simulink model "IOControls"  (R2019b)
settings: configuration reference "ConfigSet_IOControls_Reference" (kept outside this file)
model workspace (MAT data in the model file):
  SampleTime = 0.05
libraries: IOStateMachinesLib x274, SignalGeneratorsLib x1, simulink x1
(part 4 of 10)

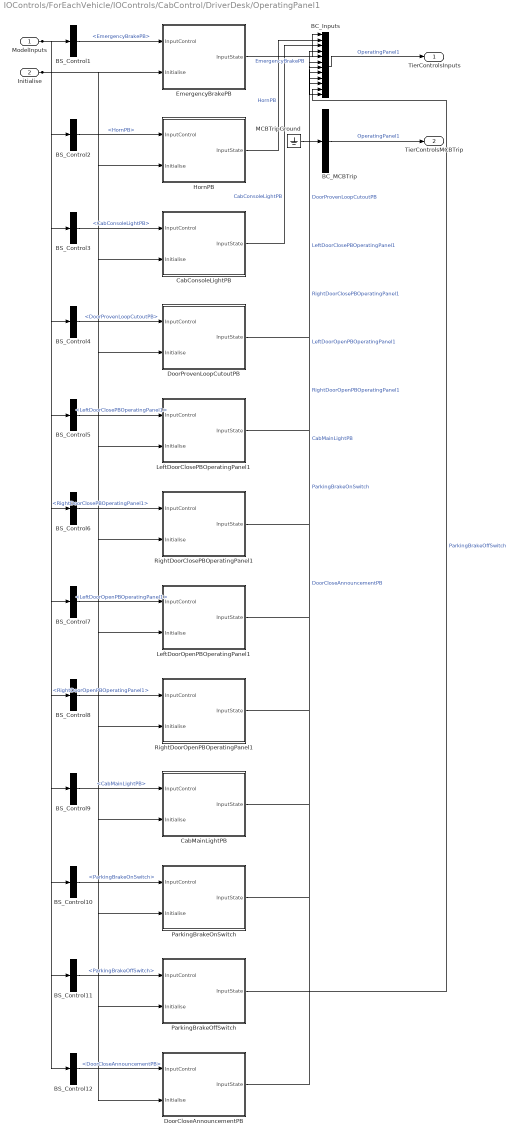
== system IOControls/ForEachVehicle/IOControls/CabControl/DriverDesk/OperatingPanel1 ==
  ModelInputs : Inport
  Initialise : Inport  Port=2
  BC_Inputs : BusCreator  Inputs=12
  BC_MCBTrip : BusCreator  Inputs=1
  BS_Control1 : BusSelector  OutputSignals=EmergencyBrakePB
  BS_Control10 : BusSelector  OutputSignals=ParkingBrakeOnSwitch
  BS_Control11 : BusSelector  OutputSignals=ParkingBrakeOffSwitch
  BS_Control12 : BusSelector  OutputSignals=DoorCloseAnnouncementPB
  BS_Control2 : BusSelector  OutputSignals=HornPB
  BS_Control3 : BusSelector  OutputSignals=CabConsoleLightPB
  BS_Control4 : BusSelector  OutputSignals=DoorProvenLoopCutoutPB
  BS_Control5 : BusSelector  OutputSignals=LeftDoorClosePBOperatingPanel1
  BS_Control6 : BusSelector  OutputSignals=RightDoorClosePBOperatingPanel1
  BS_Control7 : BusSelector  OutputSignals=LeftDoorOpenPBOperatingPanel1
  BS_Control8 : BusSelector  OutputSignals=RightDoorOpenPBOperatingPanel1
  BS_Control9 : BusSelector  OutputSignals=CabMainLightPB
  CabConsoleLightPB : Subsystem  mask{InitState=0, ControlStates=[0,1], OnStateValue=1, OffStateValue=0}
      mask prompts: InitState "Initial State"; ControlStates "Software State Values"; OnStateValue "On State Value"; OffStateValue "Off State Value"
  CabMainLightPB : Subsystem  mask{InitState=0, ControlStates=[0,1], OnStateValue=1, OffStateValue=0}
      mask prompts: InitState "Initial State"; ControlStates "Software State Values"; OnStateValue "On State Value"; OffStateValue "Off State Value"
  DoorCloseAnnouncementPB : Subsystem  mask{InitState=0, ControlStates=[0,1], OnStateValue=1, OffStateValue=0}
      mask prompts: InitState "Initial State"; ControlStates "Software State Values"; OnStateValue "On State Value"; OffStateValue "Off State Value"
  DoorProvenLoopCutoutPB : Subsystem  mask{InitState=0, ControlStates=[0,1], OnStateValue=1, OffStateValue=0}
      mask prompts: InitState "Initial State"; ControlStates "Software State Values"; OnStateValue "On State Value"; OffStateValue "Off State Value"
  EmergencyBrakePB : Subsystem  mask{InitState=0, ControlStates=[0,1], OnStateValue=1, OffStateValue=0}
      mask prompts: InitState "Initial State"; ControlStates "Software State Values"; OnStateValue "On State Value"; OffStateValue "Off State Value"
  HornPB : Subsystem  mask{InitState=0, ControlStates=[0,1], OnStateValue=1, OffStateValue=0}
      mask prompts: InitState "Initial State"; ControlStates "Software State Values"; OnStateValue "On State Value"; OffStateValue "Off State Value"
  LeftDoorClosePBOperatingPanel1 : Subsystem  mask{InitState=0, ControlStates=[0,1], OnStateValue=1, OffStateValue=0}
      mask prompts: InitState "Initial State"; ControlStates "Software State Values"; OnStateValue "On State Value"; OffStateValue "Off State Value"
  LeftDoorOpenPBOperatingPanel1 : Subsystem  mask{InitState=0, ControlStates=[0,1], OnStateValue=1, OffStateValue=0}
      mask prompts: InitState "Initial State"; ControlStates "Software State Values"; OnStateValue "On State Value"; OffStateValue "Off State Value"
  MCBTripGround : Ground
  ParkingBrakeOffSwitch : Subsystem  mask{InitState=0, ControlStates=[0,1], OnStateValue=1, OffStateValue=0}
      mask prompts: InitState "Initial State"; ControlStates "Software State Values"; OnStateValue "On State Value"; OffStateValue "Off State Value"
  ParkingBrakeOnSwitch : Subsystem  mask{InitState=0, ControlStates=[0,1], OnStateValue=1, OffStateValue=0}
      mask prompts: InitState "Initial State"; ControlStates "Software State Values"; OnStateValue "On State Value"; OffStateValue "Off State Value"
  RightDoorClosePBOperatingPanel1 : Subsystem  mask{InitState=0, ControlStates=[0,1], OnStateValue=1, OffStateValue=0}
      mask prompts: InitState "Initial State"; ControlStates "Software State Values"; OnStateValue "On State Value"; OffStateValue "Off State Value"
  RightDoorOpenPBOperatingPanel1 : Subsystem  mask{InitState=0, ControlStates=[0,1], OnStateValue=1, OffStateValue=0}
      mask prompts: InitState "Initial State"; ControlStates "Software State Values"; OnStateValue "On State Value"; OffStateValue "Off State Value"
  TierControlsInputs : Outport  VectorParamsAs1DForOutWhenUnconnected=off
  TierControlsMCBTrip : Outport  Port=2  VectorParamsAs1DForOutWhenUnconnected=off
  wires:
  MCBTripGround/1 -> BC_MCBTrip/1
  BC_MCBTrip/1 -> TierControlsMCBTrip/1  "OperatingPanel1"
  BC_Inputs/1 -> TierControlsInputs/1  "OperatingPanel1"
  ModelInputs/1 -> BS_Control1/1, BS_Control2/1, BS_Control3/1, BS_Control4/1, BS_Control5/1, BS_Control6/1, BS_Control7/1, BS_Control8/1, BS_Control9/1, BS_Control10/1, BS_Control11/1, BS_Control12/1
  BS_Control1/1 -> EmergencyBrakePB/1(InputControl)  "<EmergencyBrakePB>"
  Initialise/1 -> EmergencyBrakePB/2(Initialise), HornPB/2(Initialise), CabConsoleLightPB/2(Initialise), DoorProvenLoopCutoutPB/2(Initialise), LeftDoorClosePBOperatingPanel1/2(Initialise), RightDoorClosePBOperatingPanel1/2(Initialise), LeftDoorOpenPBOperatingPanel1/2(Initialise), RightDoorOpenPBOperatingPanel1/2(Initialise), CabMainLightPB/2(Initialise), ParkingBrakeOnSwitch/2(Initialise), ParkingBrakeOffSwitch/2(Initialise), DoorCloseAnnouncementPB/2(Initialise)
  EmergencyBrakePB/1(InputState) -> BC_Inputs/1  "EmergencyBrakePB"
  BS_Control2/1 -> HornPB/1(InputControl)  "<HornPB>"
  HornPB/1(InputState) -> BC_Inputs/2  "HornPB"
  BS_Control3/1 -> CabConsoleLightPB/1(InputControl)  "<CabConsoleLightPB>"
  CabConsoleLightPB/1(InputState) -> BC_Inputs/3  "CabConsoleLightPB"
  BS_Control4/1 -> DoorProvenLoopCutoutPB/1(InputControl)  "<DoorProvenLoopCutoutPB>"
  DoorProvenLoopCutoutPB/1(InputState) -> BC_Inputs/4  "DoorProvenLoopCutoutPB"
  BS_Control5/1 -> LeftDoorClosePBOperatingPanel1/1(InputControl)  "<LeftDoorClosePBOperatingPanel1>"
  LeftDoorClosePBOperatingPanel1/1(InputState) -> BC_Inputs/5  "LeftDoorClosePBOperatingPanel1"
  BS_Control6/1 -> RightDoorClosePBOperatingPanel1/1(InputControl)  "<RightDoorClosePBOperatingPanel1>"
  RightDoorClosePBOperatingPanel1/1(InputState) -> BC_Inputs/6  "RightDoorClosePBOperatingPanel1"
  BS_Control7/1 -> LeftDoorOpenPBOperatingPanel1/1(InputControl)  "<LeftDoorOpenPBOperatingPanel1>"
  LeftDoorOpenPBOperatingPanel1/1(InputState) -> BC_Inputs/7  "LeftDoorOpenPBOperatingPanel1"
  BS_Control8/1 -> RightDoorOpenPBOperatingPanel1/1(InputControl)  "<RightDoorOpenPBOperatingPanel1>"
  RightDoorOpenPBOperatingPanel1/1(InputState) -> BC_Inputs/8  "RightDoorOpenPBOperatingPanel1"
  BS_Control9/1 -> CabMainLightPB/1(InputControl)  "<CabMainLightPB>"
  CabMainLightPB/1(InputState) -> BC_Inputs/9  "CabMainLightPB"
  BS_Control10/1 -> ParkingBrakeOnSwitch/1(InputControl)  "<ParkingBrakeOnSwitch>"
  ParkingBrakeOnSwitch/1(InputState) -> BC_Inputs/10  "ParkingBrakeOnSwitch"
  BS_Control11/1 -> ParkingBrakeOffSwitch/1(InputControl)  "<ParkingBrakeOffSwitch>"
  ParkingBrakeOffSwitch/1(InputState) -> BC_Inputs/11  "ParkingBrakeOffSwitch"
  BS_Control12/1 -> DoorCloseAnnouncementPB/1(InputControl)  "<DoorCloseAnnouncementPB>"
  DoorCloseAnnouncementPB/1(InputState) -> BC_Inputs/12  "DoorCloseAnnouncementPB"

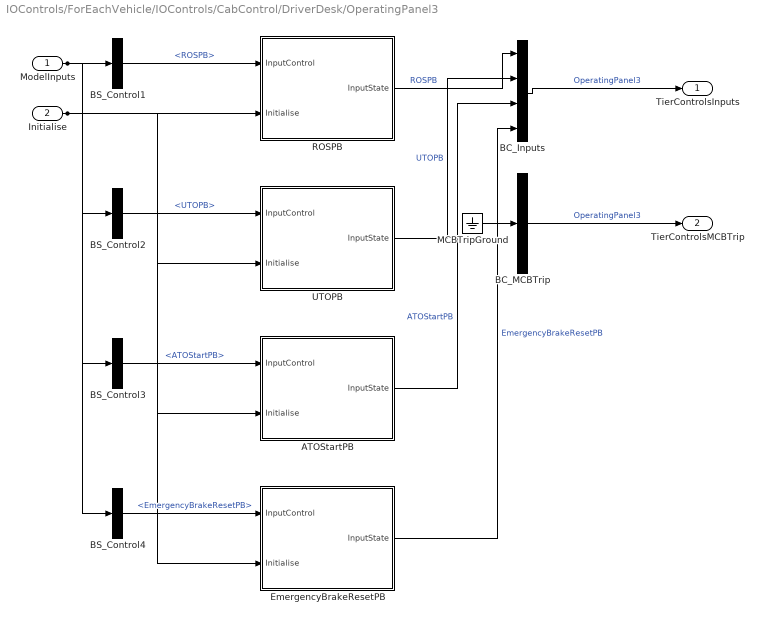
== system IOControls/ForEachVehicle/IOControls/CabControl/DriverDesk/OperatingPanel3 ==
  ModelInputs : Inport
  Initialise : Inport  Port=2
  ATOStartPB : Subsystem  mask{InitState=0, ControlStates=[0,1], OnStateValue=1, OffStateValue=0}
      mask prompts: InitState "Initial State"; ControlStates "Software State Values"; OnStateValue "On State Value"; OffStateValue "Off State Value"
  BC_Inputs : BusCreator  Inputs=4
  BC_MCBTrip : BusCreator  Inputs=1
  BS_Control1 : BusSelector  OutputSignals=ROSPB
  BS_Control2 : BusSelector  OutputSignals=UTOPB
  BS_Control3 : BusSelector  OutputSignals=ATOStartPB
  BS_Control4 : BusSelector  OutputSignals=EmergencyBrakeResetPB
  EmergencyBrakeResetPB : Subsystem  mask{InitState=0, ControlStates=[0,1], OnStateValue=1, OffStateValue=0}
      mask prompts: InitState "Initial State"; ControlStates "Software State Values"; OnStateValue "On State Value"; OffStateValue "Off State Value"
  MCBTripGround : Ground
  ROSPB : Subsystem  mask{InitState=0, ControlStates=[0,1], OnStateValue=1, OffStateValue=0}
      mask prompts: InitState "Initial State"; ControlStates "Software State Values"; OnStateValue "On State Value"; OffStateValue "Off State Value"
  UTOPB : Subsystem  mask{InitState=0, ControlStates=[0,1], OnStateValue=1, OffStateValue=0}
      mask prompts: InitState "Initial State"; ControlStates "Software State Values"; OnStateValue "On State Value"; OffStateValue "Off State Value"
  TierControlsInputs : Outport  VectorParamsAs1DForOutWhenUnconnected=off
  TierControlsMCBTrip : Outport  Port=2  VectorParamsAs1DForOutWhenUnconnected=off
  wires:
  MCBTripGround/1 -> BC_MCBTrip/1
  BC_MCBTrip/1 -> TierControlsMCBTrip/1  "OperatingPanel3"
  BC_Inputs/1 -> TierControlsInputs/1  "OperatingPanel3"
  ModelInputs/1 -> BS_Control1/1, BS_Control2/1, BS_Control3/1, BS_Control4/1
  BS_Control1/1 -> ROSPB/1(InputControl)  "<ROSPB>"
  Initialise/1 -> ROSPB/2(Initialise), UTOPB/2(Initialise), ATOStartPB/2(Initialise), EmergencyBrakeResetPB/2(Initialise)
  ROSPB/1(InputState) -> BC_Inputs/1  "ROSPB"
  BS_Control2/1 -> UTOPB/1(InputControl)  "<UTOPB>"
  UTOPB/1(InputState) -> BC_Inputs/2  "UTOPB"
  BS_Control3/1 -> ATOStartPB/1(InputControl)  "<ATOStartPB>"
  ATOStartPB/1(InputState) -> BC_Inputs/3  "ATOStartPB"
  BS_Control4/1 -> EmergencyBrakeResetPB/1(InputControl)  "<EmergencyBrakeResetPB>"
  EmergencyBrakeResetPB/1(InputState) -> BC_Inputs/4  "EmergencyBrakeResetPB"

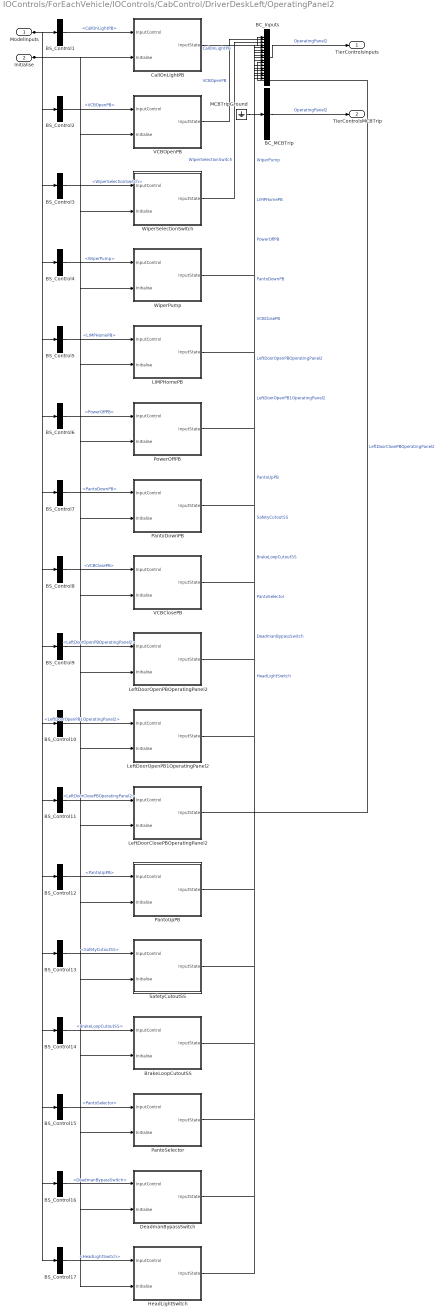
== system IOControls/ForEachVehicle/IOControls/CabControl/DriverDeskLeft/OperatingPanel2 ==
  ModelInputs : Inport
  Initialise : Inport  Port=2
  BC_Inputs : BusCreator  Inputs=17
  BC_MCBTrip : BusCreator  Inputs=1
  BS_Control1 : BusSelector  OutputSignals=CallOnLightPB
  BS_Control10 : BusSelector  OutputSignals=LeftDoorOpenPB1OperatingPanel2
  BS_Control11 : BusSelector  OutputSignals=LeftDoorClosePBOperatingPanel2
  BS_Control12 : BusSelector  OutputSignals=PantoUpPB
  BS_Control13 : BusSelector  OutputSignals=SafetyCutoutSS
  BS_Control14 : BusSelector  OutputSignals=BrakeLoopCutoutSS
  BS_Control15 : BusSelector  OutputSignals=PantoSelector
  BS_Control16 : BusSelector  OutputSignals=DeadmanBypassSwitch
  BS_Control17 : BusSelector  OutputSignals=HeadLightSwitch
  BS_Control2 : BusSelector  OutputSignals=VCBOpenPB
  BS_Control3 : BusSelector  OutputSignals=WiperSelectionSwitch
  BS_Control4 : BusSelector  OutputSignals=WiperPump
  BS_Control5 : BusSelector  OutputSignals=LIMPHomePB
  BS_Control6 : BusSelector  OutputSignals=PowerOffPB
  BS_Control7 : BusSelector  OutputSignals=PantoDownPB
  BS_Control8 : BusSelector  OutputSignals=VCBClosePB
  BS_Control9 : BusSelector  OutputSignals=LeftDoorOpenPBOperatingPanel2
  BrakeLoopCutoutSS : Subsystem  mask{InitState=0, ControlStates=[0,1], OnStateValue=1, OffStateValue=0}
      mask prompts: InitState "Initial State"; ControlStates "Software State Values"; OnStateValue "On State Value"; OffStateValue "Off State Value"
  CallOnLightPB : Subsystem  mask{InitState=0, ControlStates=[0,1], OnStateValue=1, OffStateValue=0}
      mask prompts: InitState "Initial State"; ControlStates "Software State Values"; OnStateValue "On State Value"; OffStateValue "Off State Value"
  DeadmanBypassSwitch : Subsystem  mask{InitState=0, ControlStates=[0,1], OnStateValue=1, OffStateValue=0}
      mask prompts: InitState "Initial State"; ControlStates "Software State Values"; OnStateValue "On State Value"; OffStateValue "Off State Value"
  HeadLightSwitch : Subsystem  mask{InitState=0, ControlStates=[0,1,2], OnStateValue=2, OffStateValue=0}
      mask prompts: InitState "Initial State"; ControlStates "Software State Values"; OnStateValue "On State Value"; OffStateValue "Off State Value"
  LIMPHomePB : Subsystem  mask{InitState=0, ControlStates=[0,1], OnStateValue=1, OffStateValue=0}
      mask prompts: InitState "Initial State"; ControlStates "Software State Values"; OnStateValue "On State Value"; OffStateValue "Off State Value"
  LeftDoorClosePBOperatingPanel2 : Subsystem  mask{InitState=0, ControlStates=[0,1], OnStateValue=1, OffStateValue=0}
      mask prompts: InitState "Initial State"; ControlStates "Software State Values"; OnStateValue "On State Value"; OffStateValue "Off State Value"
  LeftDoorOpenPB1OperatingPanel2 : Subsystem  mask{InitState=0, ControlStates=[0,1], OnStateValue=1, OffStateValue=0}
      mask prompts: InitState "Initial State"; ControlStates "Software State Values"; OnStateValue "On State Value"; OffStateValue "Off State Value"
  LeftDoorOpenPBOperatingPanel2 : Subsystem  mask{InitState=0, ControlStates=[0,1], OnStateValue=1, OffStateValue=0}
      mask prompts: InitState "Initial State"; ControlStates "Software State Values"; OnStateValue "On State Value"; OffStateValue "Off State Value"
  MCBTripGround : Ground
  PantoDownPB : Subsystem  mask{InitState=0, ControlStates=[0,1], OnStateValue=1, OffStateValue=0}
      mask prompts: InitState "Initial State"; ControlStates "Software State Values"; OnStateValue "On State Value"; OffStateValue "Off State Value"
  PantoSelector : Subsystem  mask{InitState=0, ControlStates=[0,1,2,3], OnStateValue=3, OffStateValue=0}
      mask prompts: InitState "Initial State"; ControlStates "Software State Values"; OnStateValue "On State Value"; OffStateValue "Off State Value"
  PantoUpPB : Subsystem  mask{InitState=0, ControlStates=[0,1], OnStateValue=1, OffStateValue=0}
      mask prompts: InitState "Initial State"; ControlStates "Software State Values"; OnStateValue "On State Value"; OffStateValue "Off State Value"
  PowerOffPB : Subsystem  mask{InitState=0, ControlStates=[0,1], OnStateValue=1, OffStateValue=0}
      mask prompts: InitState "Initial State"; ControlStates "Software State Values"; OnStateValue "On State Value"; OffStateValue "Off State Value"
  SafetyCutoutSS : Subsystem  mask{InitState=0, ControlStates=[0,1], OnStateValue=1, OffStateValue=0}
      mask prompts: InitState "Initial State"; ControlStates "Software State Values"; OnStateValue "On State Value"; OffStateValue "Off State Value"
  VCBClosePB : Subsystem  mask{InitState=0, ControlStates=[0,1], OnStateValue=1, OffStateValue=0}
      mask prompts: InitState "Initial State"; ControlStates "Software State Values"; OnStateValue "On State Value"; OffStateValue "Off State Value"
  VCBOpenPB : Subsystem  mask{InitState=0, ControlStates=[0,1], OnStateValue=1, OffStateValue=0}
      mask prompts: InitState "Initial State"; ControlStates "Software State Values"; OnStateValue "On State Value"; OffStateValue "Off State Value"
  WiperPump : Subsystem  mask{InitState=0, ControlStates=[0,1], OnStateValue=1, OffStateValue=0}
      mask prompts: InitState "Initial State"; ControlStates "Software State Values"; OnStateValue "On State Value"; OffStateValue "Off State Value"
  WiperSelectionSwitch : Subsystem  mask{InitState=0, ControlStates=[0,1,2,3], OnStateValue=3, OffStateValue=0}
      mask prompts: InitState "Initial State"; ControlStates "Software State Values"; OnStateValue "On State Value"; OffStateValue "Off State Value"
  TierControlsInputs : Outport  VectorParamsAs1DForOutWhenUnconnected=off
  TierControlsMCBTrip : Outport  Port=2  VectorParamsAs1DForOutWhenUnconnected=off
  wires:
  MCBTripGround/1 -> BC_MCBTrip/1
  BC_MCBTrip/1 -> TierControlsMCBTrip/1  "OperatingPanel2"
  BC_Inputs/1 -> TierControlsInputs/1  "OperatingPanel2"
  ModelInputs/1 -> BS_Control1/1, BS_Control2/1, BS_Control3/1, BS_Control4/1, BS_Control5/1, BS_Control6/1, BS_Control7/1, BS_Control8/1, BS_Control9/1, BS_Control10/1, BS_Control11/1, BS_Control12/1, BS_Control13/1, BS_Control14/1, BS_Control15/1, BS_Control16/1, BS_Control17/1
  BS_Control1/1 -> CallOnLightPB/1(InputControl)  "<CallOnLightPB>"
  Initialise/1 -> CallOnLightPB/2(Initialise), VCBOpenPB/2(Initialise), WiperSelectionSwitch/2(Initialise), WiperPump/2(Initialise), LIMPHomePB/2(Initialise), PowerOffPB/2(Initialise), PantoDownPB/2(Initialise), VCBClosePB/2(Initialise), LeftDoorOpenPBOperatingPanel2/2(Initialise), LeftDoorOpenPB1OperatingPanel2/2(Initialise), LeftDoorClosePBOperatingPanel2/2(Initialise), PantoUpPB/2(Initialise), SafetyCutoutSS/2(Initialise), BrakeLoopCutoutSS/2(Initialise), PantoSelector/2(Initialise), DeadmanBypassSwitch/2(Initialise), HeadLightSwitch/2(Initialise)
  CallOnLightPB/1(InputState) -> BC_Inputs/1  "CallOnLightPB"
  BS_Control2/1 -> VCBOpenPB/1(InputControl)  "<VCBOpenPB>"
  VCBOpenPB/1(InputState) -> BC_Inputs/2  "VCBOpenPB"
  BS_Control3/1 -> WiperSelectionSwitch/1(InputControl)  "<WiperSelectionSwitch>"
  WiperSelectionSwitch/1(InputState) -> BC_Inputs/3  "WiperSelectionSwitch"
  BS_Control4/1 -> WiperPump/1(InputControl)  "<WiperPump>"
  WiperPump/1(InputState) -> BC_Inputs/4  "WiperPump"
  BS_Control5/1 -> LIMPHomePB/1(InputControl)  "<LIMPHomePB>"
  LIMPHomePB/1(InputState) -> BC_Inputs/5  "LIMPHomePB"
  BS_Control6/1 -> PowerOffPB/1(InputControl)  "<PowerOffPB>"
  PowerOffPB/1(InputState) -> BC_Inputs/6  "PowerOffPB"
  BS_Control7/1 -> PantoDownPB/1(InputControl)  "<PantoDownPB>"
  PantoDownPB/1(InputState) -> BC_Inputs/7  "PantoDownPB"
  BS_Control8/1 -> VCBClosePB/1(InputControl)  "<VCBClosePB>"
  VCBClosePB/1(InputState) -> BC_Inputs/8  "VCBClosePB"
  BS_Control9/1 -> LeftDoorOpenPBOperatingPanel2/1(InputControl)  "<LeftDoorOpenPBOperatingPanel2>"
  LeftDoorOpenPBOperatingPanel2/1(InputState) -> BC_Inputs/9  "LeftDoorOpenPBOperatingPanel2"
  BS_Control10/1 -> LeftDoorOpenPB1OperatingPanel2/1(InputControl)  "<LeftDoorOpenPB1OperatingPanel2>"
  LeftDoorOpenPB1OperatingPanel2/1(InputState) -> BC_Inputs/10  "LeftDoorOpenPB1OperatingPanel2"
  BS_Control11/1 -> LeftDoorClosePBOperatingPanel2/1(InputControl)  "<LeftDoorClosePBOperatingPanel2>"
  LeftDoorClosePBOperatingPanel2/1(InputState) -> BC_Inputs/11  "LeftDoorClosePBOperatingPanel2"
  BS_Control12/1 -> PantoUpPB/1(InputControl)  "<PantoUpPB>"
  PantoUpPB/1(InputState) -> BC_Inputs/12  "PantoUpPB"
  BS_Control13/1 -> SafetyCutoutSS/1(InputControl)  "<SafetyCutoutSS>"
  SafetyCutoutSS/1(InputState) -> BC_Inputs/13  "SafetyCutoutSS"
  BS_Control14/1 -> BrakeLoopCutoutSS/1(InputControl)  "<BrakeLoopCutoutSS>"
  BrakeLoopCutoutSS/1(InputState) -> BC_Inputs/14  "BrakeLoopCutoutSS"
  BS_Control15/1 -> PantoSelector/1(InputControl)  "<PantoSelector>"
  PantoSelector/1(InputState) -> BC_Inputs/15  "PantoSelector"
  BS_Control16/1 -> DeadmanBypassSwitch/1(InputControl)  "<DeadmanBypassSwitch>"
  DeadmanBypassSwitch/1(InputState) -> BC_Inputs/16  "DeadmanBypassSwitch"
  BS_Control17/1 -> HeadLightSwitch/1(InputControl)  "<HeadLightSwitch>"
  HeadLightSwitch/1(InputState) -> BC_Inputs/17  "HeadLightSwitch"

== system IOControls/ForEachVehicle/IOControls/CabControl/DriverDeskLeft/OperatingPanel4 ==
  ModelInputs : Inport
  Initialise : Inport  Port=2
  BC_Inputs : BusCreator  Inputs=1
  BC_MCBTrip : BusCreator  Inputs=1
  InitialiseTerminator : Terminator
  InputsGround : Ground
  MCBTripGround : Ground
  ModelInputsTerminator : Terminator
  TierControlsInputs : Outport  VectorParamsAs1DForOutWhenUnconnected=off
  TierControlsMCBTrip : Outport  Port=2  VectorParamsAs1DForOutWhenUnconnected=off
  wires:
  MCBTripGround/1 -> BC_MCBTrip/1
  InputsGround/1 -> BC_Inputs/1
  Initialise/1 -> InitialiseTerminator/1
  ModelInputs/1 -> ModelInputsTerminator/1
  BC_MCBTrip/1 -> TierControlsMCBTrip/1  "OperatingPanel4"
  BC_Inputs/1 -> TierControlsInputs/1  "OperatingPanel4"

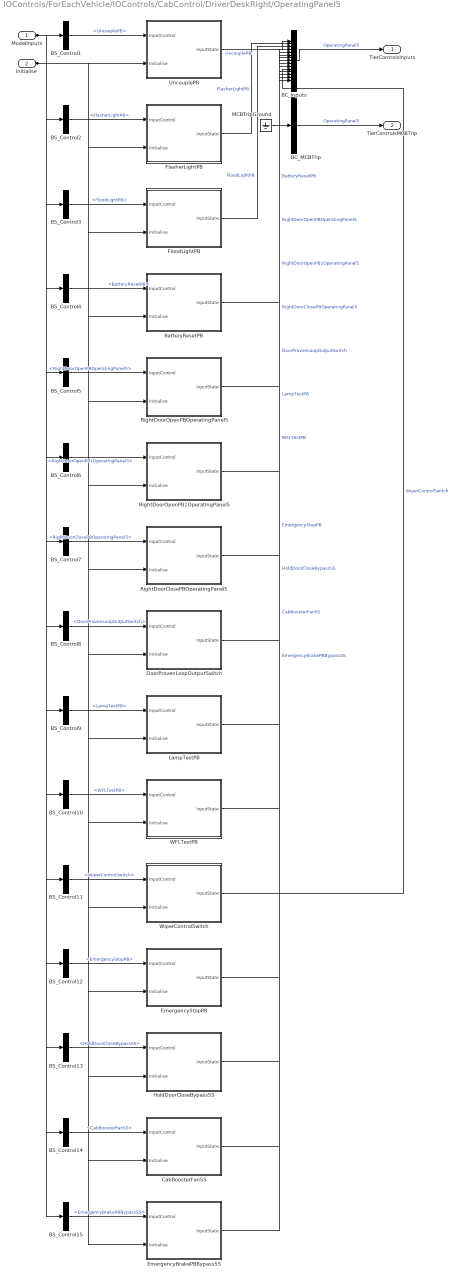
== system IOControls/ForEachVehicle/IOControls/CabControl/DriverDeskRight/OperatingPanel5 ==
  ModelInputs : Inport
  Initialise : Inport  Port=2
  BC_Inputs : BusCreator  Inputs=15
  BC_MCBTrip : BusCreator  Inputs=1
  BS_Control1 : BusSelector  OutputSignals=UncouplePB
  BS_Control10 : BusSelector  OutputSignals=WFLTestPB
  BS_Control11 : BusSelector  OutputSignals=WiperControlSwitch
  BS_Control12 : BusSelector  OutputSignals=EmergencyStopPB
  BS_Control13 : BusSelector  OutputSignals=HoldDoorCloseBypassSS
  BS_Control14 : BusSelector  OutputSignals=CabBoosterFanSS
  BS_Control15 : BusSelector  OutputSignals=EmergencyBrakePBBypassSS
  BS_Control2 : BusSelector  OutputSignals=FlasherLightPB
  BS_Control3 : BusSelector  OutputSignals=FloodLightPB
  BS_Control4 : BusSelector  OutputSignals=BatteryResetPB
  BS_Control5 : BusSelector  OutputSignals=RightDoorOpenPBOperatingPanel5
  BS_Control6 : BusSelector  OutputSignals=RightDoorOpenPB1OperatingPanel5
  BS_Control7 : BusSelector  OutputSignals=RightDoorClosePBOperatingPanel5
  BS_Control8 : BusSelector  OutputSignals=DoorProvenLoopOutputSwitch
  BS_Control9 : BusSelector  OutputSignals=LampTestPB
  BatteryResetPB : Subsystem  mask{InitState=0, ControlStates=[0,1], OnStateValue=1, OffStateValue=0}
      mask prompts: InitState "Initial State"; ControlStates "Software State Values"; OnStateValue "On State Value"; OffStateValue "Off State Value"
  CabBoosterFanSS : Subsystem  mask{InitState=0, ControlStates=[0,1,2], OnStateValue=2, OffStateValue=0}
      mask prompts: InitState "Initial State"; ControlStates "Software State Values"; OnStateValue "On State Value"; OffStateValue "Off State Value"
  DoorProvenLoopOutputSwitch : Subsystem  mask{InitState=0, ControlStates=[0,1], OnStateValue=1, OffStateValue=0}
      mask prompts: InitState "Initial State"; ControlStates "Software State Values"; OnStateValue "On State Value"; OffStateValue "Off State Value"
  EmergencyBrakePBBypassSS : Subsystem  mask{InitState=0, ControlStates=[0,1], OnStateValue=1, OffStateValue=0}
      mask prompts: InitState "Initial State"; ControlStates "Software State Values"; OnStateValue "On State Value"; OffStateValue "Off State Value"
  EmergencyStopPB : Subsystem  mask{InitState=0, ControlStates=[0,1], OnStateValue=1, OffStateValue=0}
      mask prompts: InitState "Initial State"; ControlStates "Software State Values"; OnStateValue "On State Value"; OffStateValue "Off State Value"
  FlasherLightPB : Subsystem  mask{InitState=0, ControlStates=[0,1], OnStateValue=1, OffStateValue=0}
      mask prompts: InitState "Initial State"; ControlStates "Software State Values"; OnStateValue "On State Value"; OffStateValue "Off State Value"
  FloodLightPB : Subsystem  mask{InitState=0, ControlStates=[0,1], OnStateValue=1, OffStateValue=0}
      mask prompts: InitState "Initial State"; ControlStates "Software State Values"; OnStateValue "On State Value"; OffStateValue "Off State Value"
  HoldDoorCloseBypassSS : Subsystem  mask{InitState=0, ControlStates=[0,1,2], OnStateValue=2, OffStateValue=0}
      mask prompts: InitState "Initial State"; ControlStates "Software State Values"; OnStateValue "On State Value"; OffStateValue "Off State Value"
  LampTestPB : Subsystem  mask{InitState=0, ControlStates=[0,1], OnStateValue=1, OffStateValue=0}
      mask prompts: InitState "Initial State"; ControlStates "Software State Values"; OnStateValue "On State Value"; OffStateValue "Off State Value"
  MCBTripGround : Ground
  RightDoorClosePBOperatingPanel5 : Subsystem  mask{InitState=0, ControlStates=[0,1], OnStateValue=1, OffStateValue=0}
      mask prompts: InitState "Initial State"; ControlStates "Software State Values"; OnStateValue "On State Value"; OffStateValue "Off State Value"
  RightDoorOpenPB1OperatingPanel5 : Subsystem  mask{InitState=0, ControlStates=[0,1], OnStateValue=1, OffStateValue=0}
      mask prompts: InitState "Initial State"; ControlStates "Software State Values"; OnStateValue "On State Value"; OffStateValue "Off State Value"
  RightDoorOpenPBOperatingPanel5 : Subsystem  mask{InitState=0, ControlStates=[0,1], OnStateValue=1, OffStateValue=0}
      mask prompts: InitState "Initial State"; ControlStates "Software State Values"; OnStateValue "On State Value"; OffStateValue "Off State Value"
  UncouplePB : Subsystem  mask{InitState=0, ControlStates=[0,1], OnStateValue=1, OffStateValue=0}
      mask prompts: InitState "Initial State"; ControlStates "Software State Values"; OnStateValue "On State Value"; OffStateValue "Off State Value"
  WFLTestPB : Subsystem  mask{InitState=0, ControlStates=[0,1], OnStateValue=1, OffStateValue=0}
      mask prompts: InitState "Initial State"; ControlStates "Software State Values"; OnStateValue "On State Value"; OffStateValue "Off State Value"
  WiperControlSwitch : Subsystem  mask{InitState=0, ControlStates=[-1,0,1,2], OnStateValue=2, OffStateValue=1}
      mask prompts: InitState "Initial State"; ControlStates "Software State Values"; OnStateValue "On State Value"; OffStateValue "Off State Value"
  TierControlsInputs : Outport  VectorParamsAs1DForOutWhenUnconnected=off
  TierControlsMCBTrip : Outport  Port=2  VectorParamsAs1DForOutWhenUnconnected=off
  wires:
  MCBTripGround/1 -> BC_MCBTrip/1
  BC_MCBTrip/1 -> TierControlsMCBTrip/1  "OperatingPanel5"
  BC_Inputs/1 -> TierControlsInputs/1  "OperatingPanel5"
  ModelInputs/1 -> BS_Control1/1, BS_Control2/1, BS_Control3/1, BS_Control4/1, BS_Control5/1, BS_Control6/1, BS_Control7/1, BS_Control8/1, BS_Control9/1, BS_Control10/1, BS_Control11/1, BS_Control12/1, BS_Control13/1, BS_Control14/1, BS_Control15/1
  BS_Control1/1 -> UncouplePB/1(InputControl)  "<UncouplePB>"
  Initialise/1 -> UncouplePB/2(Initialise), FlasherLightPB/2(Initialise), FloodLightPB/2(Initialise), BatteryResetPB/2(Initialise), RightDoorOpenPBOperatingPanel5/2(Initialise), RightDoorOpenPB1OperatingPanel5/2(Initialise), RightDoorClosePBOperatingPanel5/2(Initialise), DoorProvenLoopOutputSwitch/2(Initialise), LampTestPB/2(Initialise), WFLTestPB/2(Initialise), WiperControlSwitch/2(Initialise), EmergencyStopPB/2(Initialise), HoldDoorCloseBypassSS/2(Initialise), CabBoosterFanSS/2(Initialise), EmergencyBrakePBBypassSS/2(Initialise)
  UncouplePB/1(InputState) -> BC_Inputs/1  "UncouplePB"
  BS_Control2/1 -> FlasherLightPB/1(InputControl)  "<FlasherLightPB>"
  FlasherLightPB/1(InputState) -> BC_Inputs/2  "FlasherLightPB"
  BS_Control3/1 -> FloodLightPB/1(InputControl)  "<FloodLightPB>"
  FloodLightPB/1(InputState) -> BC_Inputs/3  "FloodLightPB"
  BS_Control4/1 -> BatteryResetPB/1(InputControl)  "<BatteryResetPB>"
  BatteryResetPB/1(InputState) -> BC_Inputs/4  "BatteryResetPB"
  BS_Control5/1 -> RightDoorOpenPBOperatingPanel5/1(InputControl)  "<RightDoorOpenPBOperatingPanel5>"
  RightDoorOpenPBOperatingPanel5/1(InputState) -> BC_Inputs/5  "RightDoorOpenPBOperatingPanel5"
  BS_Control6/1 -> RightDoorOpenPB1OperatingPanel5/1(InputControl)  "<RightDoorOpenPB1OperatingPanel5>"
  RightDoorOpenPB1OperatingPanel5/1(InputState) -> BC_Inputs/6  "RightDoorOpenPB1OperatingPanel5"
  BS_Control7/1 -> RightDoorClosePBOperatingPanel5/1(InputControl)  "<RightDoorClosePBOperatingPanel5>"
  RightDoorClosePBOperatingPanel5/1(InputState) -> BC_Inputs/7  "RightDoorClosePBOperatingPanel5"
  BS_Control8/1 -> DoorProvenLoopOutputSwitch/1(InputControl)  "<DoorProvenLoopOutputSwitch>"
  DoorProvenLoopOutputSwitch/1(InputState) -> BC_Inputs/8  "DoorProvenLoopOutputSwitch"
  BS_Control9/1 -> LampTestPB/1(InputControl)  "<LampTestPB>"
  LampTestPB/1(InputState) -> BC_Inputs/9  "LampTestPB"
  BS_Control10/1 -> WFLTestPB/1(InputControl)  "<WFLTestPB>"
  WFLTestPB/1(InputState) -> BC_Inputs/10  "WFLTestPB"
  BS_Control11/1 -> WiperControlSwitch/1(InputControl)  "<WiperControlSwitch>"
  WiperControlSwitch/1(InputState) -> BC_Inputs/11  "WiperControlSwitch"
  BS_Control12/1 -> EmergencyStopPB/1(InputControl)  "<EmergencyStopPB>"
  EmergencyStopPB/1(InputState) -> BC_Inputs/12  "EmergencyStopPB"
  BS_Control13/1 -> HoldDoorCloseBypassSS/1(InputControl)  "<HoldDoorCloseBypassSS>"
  HoldDoorCloseBypassSS/1(InputState) -> BC_Inputs/13  "HoldDoorCloseBypassSS"
  BS_Control14/1 -> CabBoosterFanSS/1(InputControl)  "<CabBoosterFanSS>"
  CabBoosterFanSS/1(InputState) -> BC_Inputs/14  "CabBoosterFanSS"
  BS_Control15/1 -> EmergencyBrakePBBypassSS/1(InputControl)  "<EmergencyBrakePBBypassSS>"
  EmergencyBrakePBBypassSS/1(InputState) -> BC_Inputs/15  "EmergencyBrakePBBypassSS"

== system IOControls/ForEachVehicle/IOControls/CabControl/DriversSideCovingPanel/CabEEDLeft ==
  note: States:
      | Normal
      | Unlock
  InputControl : Inport  OutDataTypeStr=Bus: BD_IOControls_In_InputControl
  Initialise : Inport  Port=2
  Bus Selector : BusSelector  OutputSignals=Value,Mode,InitVal,InternalRequest,Inhibit
  CabEEDLeft-Momentary : IOStateMachinesLib/Momentary  InitSource=internal  InitState=InitState
      settings: SourceProductName=IO State Machines
  InputState : Outport  VectorParamsAs1DForOutWhenUnconnected=off
  wires:
  Initialise/1 -> CabEEDLeft-Momentary/4
  CabEEDLeft-Momentary/1 -> InputState/1
  Bus Selector/5 -> CabEEDLeft-Momentary/6  "<Inhibit>"
  Bus Selector/4 -> CabEEDLeft-Momentary/5  "<InternalRequest>"
  Bus Selector/3 -> CabEEDLeft-Momentary/3  "<InitVal>"
  Bus Selector/2 -> CabEEDLeft-Momentary/2  "<Mode>"
  Bus Selector/1 -> CabEEDLeft-Momentary/1  "<Value>"
  InputControl/1 -> Bus Selector/1

== system IOControls/ForEachVehicle/IOControls/CabControl/EmergencyDoor/DoorWinder ==
  note: States:
      | Do Nothing
      | int1
      | int2
      | int3
      | int4
      | int5
      | int6
      | int7
      | int8
      | int9
      | int10
      | int11
      | Wind
  InputControl : Inport  OutDataTypeStr=Bus: BD_IOControls_In_InputControl
  Initialise : Inport  Port=2
  Bus Selector : BusSelector  OutputSignals=Value,Mode,InitVal,InternalRequest,Inhibit
  DoorWinder-Rotary : IOStateMachinesLib/Rotary  InitSource=internal  InitState=InitState  ControlStates=ControlStates
      settings: SourceProductName=IO State Machines
  InputState : Outport  VectorParamsAs1DForOutWhenUnconnected=off
  wires:
  Initialise/1 -> DoorWinder-Rotary/4
  DoorWinder-Rotary/1 -> InputState/1
  Bus Selector/5 -> DoorWinder-Rotary/6  "<Inhibit>"
  Bus Selector/4 -> DoorWinder-Rotary/5  "<InternalRequest>"
  Bus Selector/3 -> DoorWinder-Rotary/3  "<InitVal>"
  Bus Selector/2 -> DoorWinder-Rotary/2  "<Mode>"
  Bus Selector/1 -> DoorWinder-Rotary/1  "<Value>"
  InputControl/1 -> Bus Selector/1

== system IOControls/ForEachVehicle/IOControls/CabControl/EmergencyDoor/DummyCover ==
  note: States:
      | Applied
      | Removed
  InputControl : Inport  OutDataTypeStr=Bus: BD_IOControls_In_InputControl
  Initialise : Inport  Port=2
  Bus Selector : BusSelector  OutputSignals=Value,Mode,InitVal,InternalRequest,Inhibit
  DummyCover-Toggle : IOStateMachinesLib/Toggle  InitSource=internal  InitState=InitState  OffStateValue=OffStateValue  OnStateValue=OnStateValue
      settings: SourceProductName=IO State Machines
  InputState : Outport  VectorParamsAs1DForOutWhenUnconnected=off
  wires:
  Initialise/1 -> DummyCover-Toggle/4
  DummyCover-Toggle/1 -> InputState/1
  Bus Selector/5 -> DummyCover-Toggle/6  "<Inhibit>"
  Bus Selector/4 -> DummyCover-Toggle/5  "<InternalRequest>"
  Bus Selector/3 -> DummyCover-Toggle/3  "<InitVal>"
  Bus Selector/2 -> DummyCover-Toggle/2  "<Mode>"
  Bus Selector/1 -> DummyCover-Toggle/1  "<Value>"
  InputControl/1 -> Bus Selector/1

== system IOControls/ForEachVehicle/IOControls/CabControl/EmergencyDoor/EmergencyDoorGasSpring ==
  note: States:
      | Locked
      | unlocked
  InputControl : Inport  OutDataTypeStr=Bus: BD_IOControls_In_InputControl
  Initialise : Inport  Port=2
  Bus Selector : BusSelector  OutputSignals=Value,Mode,InitVal,InternalRequest,Inhibit
  EmergencyDoorGasSpring-Toggle : IOStateMachinesLib/Toggle  InitSource=internal  InitState=InitState  OffStateValue=OffStateValue  OnStateValue=OnStateValue
      settings: SourceProductName=IO State Machines
  InputState : Outport  VectorParamsAs1DForOutWhenUnconnected=off
  wires:
  Initialise/1 -> EmergencyDoorGasSpring-Toggle/4
  EmergencyDoorGasSpring-Toggle/1 -> InputState/1
  Bus Selector/5 -> EmergencyDoorGasSpring-Toggle/6  "<Inhibit>"
  Bus Selector/4 -> EmergencyDoorGasSpring-Toggle/5  "<InternalRequest>"
  Bus Selector/3 -> EmergencyDoorGasSpring-Toggle/3  "<InitVal>"
  Bus Selector/2 -> EmergencyDoorGasSpring-Toggle/2  "<Mode>"
  Bus Selector/1 -> EmergencyDoorGasSpring-Toggle/1  "<Value>"
  InputControl/1 -> Bus Selector/1

== system IOControls/ForEachVehicle/IOControls/CabControl/EmergencyDoor/LargeHandle ==
  note: States:
      | Stowed
      | Applied
  InputControl : Inport  OutDataTypeStr=Bus: BD_IOControls_In_InputControl
  Initialise : Inport  Port=2
  Bus Selector : BusSelector  OutputSignals=Value,Mode,InitVal,InternalRequest,Inhibit
  LargeHandle-Toggle : IOStateMachinesLib/Toggle  InitSource=internal  InitState=InitState  OffStateValue=OffStateValue  OnStateValue=OnStateValue
      settings: SourceProductName=IO State Machines
  InputState : Outport  VectorParamsAs1DForOutWhenUnconnected=off
  wires:
  Initialise/1 -> LargeHandle-Toggle/4
  LargeHandle-Toggle/1 -> InputState/1
  Bus Selector/5 -> LargeHandle-Toggle/6  "<Inhibit>"
  Bus Selector/4 -> LargeHandle-Toggle/5  "<InternalRequest>"
  Bus Selector/3 -> LargeHandle-Toggle/3  "<InitVal>"
  Bus Selector/2 -> LargeHandle-Toggle/2  "<Mode>"
  Bus Selector/1 -> LargeHandle-Toggle/1  "<Value>"
  InputControl/1 -> Bus Selector/1

== system IOControls/ForEachVehicle/IOControls/CabControl/EmergencyDoor/RampCover ==
  note: States:
      | Closed
      | Open
  InputControl : Inport  OutDataTypeStr=Bus: BD_IOControls_In_InputControl
  Initialise : Inport  Port=2
  Bus Selector : BusSelector  OutputSignals=Value,Mode,InitVal,InternalRequest,Inhibit
  RampCover-Toggle : IOStateMachinesLib/Toggle  InitSource=internal  InitState=InitState  OffStateValue=OffStateValue  OnStateValue=OnStateValue
      settings: SourceProductName=IO State Machines
  InputState : Outport  VectorParamsAs1DForOutWhenUnconnected=off
  wires:
  Initialise/1 -> RampCover-Toggle/4
  RampCover-Toggle/1 -> InputState/1
  Bus Selector/5 -> RampCover-Toggle/6  "<Inhibit>"
  Bus Selector/4 -> RampCover-Toggle/5  "<InternalRequest>"
  Bus Selector/3 -> RampCover-Toggle/3  "<InitVal>"
  Bus Selector/2 -> RampCover-Toggle/2  "<Mode>"
  Bus Selector/1 -> RampCover-Toggle/1  "<Value>"
  InputControl/1 -> Bus Selector/1

== system IOControls/ForEachVehicle/IOControls/CabControl/EmergencyDoor/RampCoverLockingLever ==
  note: States:
      | Close
      | Open
  InputControl : Inport  OutDataTypeStr=Bus: BD_IOControls_In_InputControl
  Initialise : Inport  Port=2
  Bus Selector : BusSelector  OutputSignals=Value,Mode,InitVal,InternalRequest,Inhibit
  RampCoverLockingLever-Toggle : IOStateMachinesLib/Toggle  InitSource=internal  InitState=InitState  OffStateValue=OffStateValue  OnStateValue=OnStateValue
      settings: SourceProductName=IO State Machines
  InputState : Outport  VectorParamsAs1DForOutWhenUnconnected=off
  wires:
  Initialise/1 -> RampCoverLockingLever-Toggle/4
  RampCoverLockingLever-Toggle/1 -> InputState/1
  Bus Selector/5 -> RampCoverLockingLever-Toggle/6  "<Inhibit>"
  Bus Selector/4 -> RampCoverLockingLever-Toggle/5  "<InternalRequest>"
  Bus Selector/3 -> RampCoverLockingLever-Toggle/3  "<InitVal>"
  Bus Selector/2 -> RampCoverLockingLever-Toggle/2  "<Mode>"
  Bus Selector/1 -> RampCoverLockingLever-Toggle/1  "<Value>"
  InputControl/1 -> Bus Selector/1

== system IOControls/ForEachVehicle/IOControls/CabControl/EmergencyDoor/RampEndSupport ==
  note: States:
      | Closed
      | Open
  InputControl : Inport  OutDataTypeStr=Bus: BD_IOControls_In_InputControl
  Initialise : Inport  Port=2
  Bus Selector : BusSelector  OutputSignals=Value,Mode,InitVal,InternalRequest,Inhibit
  RampEndSupport-Toggle : IOStateMachinesLib/Toggle  InitSource=internal  InitState=InitState  OffStateValue=OffStateValue  OnStateValue=OnStateValue
      settings: SourceProductName=IO State Machines
  InputState : Outport  VectorParamsAs1DForOutWhenUnconnected=off
  wires:
  Initialise/1 -> RampEndSupport-Toggle/4
  RampEndSupport-Toggle/1 -> InputState/1
  Bus Selector/5 -> RampEndSupport-Toggle/6  "<Inhibit>"
  Bus Selector/4 -> RampEndSupport-Toggle/5  "<InternalRequest>"
  Bus Selector/3 -> RampEndSupport-Toggle/3  "<InitVal>"
  Bus Selector/2 -> RampEndSupport-Toggle/2  "<Mode>"
  Bus Selector/1 -> RampEndSupport-Toggle/1  "<Value>"
  InputControl/1 -> Bus Selector/1

== system IOControls/ForEachVehicle/IOControls/CabControl/EmergencyDoor/RampHandle ==
  note: States:
      | Not Pushed
      | Pushed
  InputControl : Inport  OutDataTypeStr=Bus: BD_IOControls_In_InputControl
  Initialise : Inport  Port=2
  Bus Selector : BusSelector  OutputSignals=Value,Mode,InitVal,InternalRequest,Inhibit
  RampHandle-Toggle : IOStateMachinesLib/Toggle  InitSource=internal  InitState=InitState  OffStateValue=OffStateValue  OnStateValue=OnStateValue
      settings: SourceProductName=IO State Machines
  InputState : Outport  VectorParamsAs1DForOutWhenUnconnected=off
  wires:
  Initialise/1 -> RampHandle-Toggle/4
  RampHandle-Toggle/1 -> InputState/1
  Bus Selector/5 -> RampHandle-Toggle/6  "<Inhibit>"
  Bus Selector/4 -> RampHandle-Toggle/5  "<InternalRequest>"
  Bus Selector/3 -> RampHandle-Toggle/3  "<InitVal>"
  Bus Selector/2 -> RampHandle-Toggle/2  "<Mode>"
  Bus Selector/1 -> RampHandle-Toggle/1  "<Value>"
  InputControl/1 -> Bus Selector/1

== system IOControls/ForEachVehicle/IOControls/CabControl/EmergencyDoor/RampMiddleSupport ==
  note: States:
      | Closed
      | Open
  InputControl : Inport  OutDataTypeStr=Bus: BD_IOControls_In_InputControl
  Initialise : Inport  Port=2
  Bus Selector : BusSelector  OutputSignals=Value,Mode,InitVal,InternalRequest,Inhibit
  RampMiddleSupport-Toggle : IOStateMachinesLib/Toggle  InitSource=internal  InitState=InitState  OffStateValue=OffStateValue  OnStateValue=OnStateValue
      settings: SourceProductName=IO State Machines
  InputState : Outport  VectorParamsAs1DForOutWhenUnconnected=off
  wires:
  Initialise/1 -> RampMiddleSupport-Toggle/4
  RampMiddleSupport-Toggle/1 -> InputState/1
  Bus Selector/5 -> RampMiddleSupport-Toggle/6  "<Inhibit>"
  Bus Selector/4 -> RampMiddleSupport-Toggle/5  "<InternalRequest>"
  Bus Selector/3 -> RampMiddleSupport-Toggle/3  "<InitVal>"
  Bus Selector/2 -> RampMiddleSupport-Toggle/2  "<Mode>"
  Bus Selector/1 -> RampMiddleSupport-Toggle/1  "<Value>"
  InputControl/1 -> Bus Selector/1

== system IOControls/ForEachVehicle/IOControls/CabControl/EmergencyDoor/RampWinder ==
  note: States:
      | Do Nothing
      | int1
      | int2
      | int3
      | int4
      | int5
      | int6
      | int7
      | int8
      | int9
      | int10
      | int11
      | Wind
  InputControl : Inport  OutDataTypeStr=Bus: BD_IOControls_In_InputControl
  Initialise : Inport  Port=2
  Bus Selector : BusSelector  OutputSignals=Value,Mode,InitVal,InternalRequest,Inhibit
  RampWinder-Rotary : IOStateMachinesLib/Rotary  InitSource=internal  InitState=InitState  ControlStates=ControlStates
      settings: SourceProductName=IO State Machines
  InputState : Outport  VectorParamsAs1DForOutWhenUnconnected=off
  wires:
  Initialise/1 -> RampWinder-Rotary/4
  RampWinder-Rotary/1 -> InputState/1
  Bus Selector/5 -> RampWinder-Rotary/6  "<Inhibit>"
  Bus Selector/4 -> RampWinder-Rotary/5  "<InternalRequest>"
  Bus Selector/3 -> RampWinder-Rotary/3  "<InitVal>"
  Bus Selector/2 -> RampWinder-Rotary/2  "<Mode>"
  Bus Selector/1 -> RampWinder-Rotary/1  "<Value>"
  InputControl/1 -> Bus Selector/1

== system IOControls/ForEachVehicle/IOControls/CabControl/EmergencyDoor/SafetyCover ==
  note: States:
      | Normal
      | Broken
  InputControl : Inport  OutDataTypeStr=Bus: BD_IOControls_In_InputControl
  Initialise : Inport  Port=2
  Bus Selector : BusSelector  OutputSignals=Value,Mode,InitVal,InternalRequest,Inhibit
  SafetyCover-Toggle : IOStateMachinesLib/Toggle  InitSource=internal  InitState=InitState  OffStateValue=OffStateValue  OnStateValue=OnStateValue
      settings: SourceProductName=IO State Machines
  InputState : Outport  VectorParamsAs1DForOutWhenUnconnected=off
  wires:
  Initialise/1 -> SafetyCover-Toggle/4
  SafetyCover-Toggle/1 -> InputState/1
  Bus Selector/5 -> SafetyCover-Toggle/6  "<Inhibit>"
  Bus Selector/4 -> SafetyCover-Toggle/5  "<InternalRequest>"
  Bus Selector/3 -> SafetyCover-Toggle/3  "<InitVal>"
  Bus Selector/2 -> SafetyCover-Toggle/2  "<Mode>"
  Bus Selector/1 -> SafetyCover-Toggle/1  "<Value>"
  InputControl/1 -> Bus Selector/1

== system IOControls/ForEachVehicle/IOControls/CabControl/EmergencyDoor/SmallHandle ==
  note: States:
      | Stowed
      | Applied
  InputControl : Inport  OutDataTypeStr=Bus: BD_IOControls_In_InputControl
  Initialise : Inport  Port=2
  Bus Selector : BusSelector  OutputSignals=Value,Mode,InitVal,InternalRequest,Inhibit
  SmallHandle-Toggle : IOStateMachinesLib/Toggle  InitSource=internal  InitState=InitState  OffStateValue=OffStateValue  OnStateValue=OnStateValue
      settings: SourceProductName=IO State Machines
  InputState : Outport  VectorParamsAs1DForOutWhenUnconnected=off
  wires:
  Initialise/1 -> SmallHandle-Toggle/4
  SmallHandle-Toggle/1 -> InputState/1
  Bus Selector/5 -> SmallHandle-Toggle/6  "<Inhibit>"
  Bus Selector/4 -> SmallHandle-Toggle/5  "<InternalRequest>"
  Bus Selector/3 -> SmallHandle-Toggle/3  "<InitVal>"
  Bus Selector/2 -> SmallHandle-Toggle/2  "<Mode>"
  Bus Selector/1 -> SmallHandle-Toggle/1  "<Value>"
  InputControl/1 -> Bus Selector/1

== system IOControls/ForEachVehicle/IOControls/CabControl/EmergencyDoor/WinderHandlesAccessCover ==
  note: States:
      | Closed
      | Open
  InputControl : Inport  OutDataTypeStr=Bus: BD_IOControls_In_InputControl
  Initialise : Inport  Port=2
  Bus Selector : BusSelector  OutputSignals=Value,Mode,InitVal,InternalRequest,Inhibit
  WinderHandlesAccessCover-Toggle : IOStateMachinesLib/Toggle  InitSource=internal  InitState=InitState  OffStateValue=OffStateValue  OnStateValue=OnStateValue
      settings: SourceProductName=IO State Machines
  InputState : Outport  VectorParamsAs1DForOutWhenUnconnected=off
  wires:
  Initialise/1 -> WinderHandlesAccessCover-Toggle/4
  WinderHandlesAccessCover-Toggle/1 -> InputState/1
  Bus Selector/5 -> WinderHandlesAccessCover-Toggle/6  "<Inhibit>"
  Bus Selector/4 -> WinderHandlesAccessCover-Toggle/5  "<InternalRequest>"
  Bus Selector/3 -> WinderHandlesAccessCover-Toggle/3  "<InitVal>"
  Bus Selector/2 -> WinderHandlesAccessCover-Toggle/2  "<Mode>"
  Bus Selector/1 -> WinderHandlesAccessCover-Toggle/1  "<Value>"
  InputControl/1 -> Bus Selector/1

== system IOControls/ForEachVehicle/IOControls/CabControl/Non-driversSideCovingPanel/CabEEDRight ==
  note: States:
      | Normal
      | Unlock
  InputControl : Inport  OutDataTypeStr=Bus: BD_IOControls_In_InputControl
  Initialise : Inport  Port=2
  Bus Selector : BusSelector  OutputSignals=Value,Mode,InitVal,InternalRequest,Inhibit
  CabEEDRight-Momentary : IOStateMachinesLib/Momentary  InitSource=internal  InitState=InitState
      settings: SourceProductName=IO State Machines
  InputState : Outport  VectorParamsAs1DForOutWhenUnconnected=off
  wires:
  Initialise/1 -> CabEEDRight-Momentary/4
  CabEEDRight-Momentary/1 -> InputState/1
  Bus Selector/5 -> CabEEDRight-Momentary/6  "<Inhibit>"
  Bus Selector/4 -> CabEEDRight-Momentary/5  "<InternalRequest>"
  Bus Selector/3 -> CabEEDRight-Momentary/3  "<InitVal>"
  Bus Selector/2 -> CabEEDRight-Momentary/2  "<Mode>"
  Bus Selector/1 -> CabEEDRight-Momentary/1  "<Value>"
  InputControl/1 -> Bus Selector/1

== system IOControls/ForEachVehicle/IOControls/Non-CabControl/CircuitBreakersofEDB/AC1CB ==
  note: States:
      | Tripped
      | Set
  MCBControl : Inport  OutDataTypeStr=Bus: BD_IOControls_In_MCBControl
  Initialise : Inport  Port=2
  AC1CB-MCB : IOStateMachinesLib/MCB  InitSource=internal  InitState=InitState  OffStateValue=OffStateValue  OnStateValue=OnStateValue
      settings: SourceProductName=IO State Machines
  Bus Selector : BusSelector  OutputSignals=Value,Mode,InitVal,InternalRequest,Inhibit,TripRequest
  InputState : Outport  VectorParamsAs1DForOutWhenUnconnected=off
  MCBTripState : Outport  Port=2  VectorParamsAs1DForOutWhenUnconnected=off
  wires:
  AC1CB-MCB/2 -> MCBTripState/1
  Bus Selector/6 -> AC1CB-MCB/7  "<TripRequest>"
  MCBControl/1 -> Bus Selector/1
  Bus Selector/1 -> AC1CB-MCB/1  "<Value>"
  Bus Selector/2 -> AC1CB-MCB/2  "<Mode>"
  Bus Selector/3 -> AC1CB-MCB/3  "<InitVal>"
  Bus Selector/4 -> AC1CB-MCB/5  "<InternalRequest>"
  Bus Selector/5 -> AC1CB-MCB/6  "<Inhibit>"
  AC1CB-MCB/1 -> InputState/1
  Initialise/1 -> AC1CB-MCB/4

== system IOControls/ForEachVehicle/IOControls/Non-CabControl/CircuitBreakersofEDB/AC2CB ==
  note: States:
      | Tripped
      | Set
  MCBControl : Inport  OutDataTypeStr=Bus: BD_IOControls_In_MCBControl
  Initialise : Inport  Port=2
  AC2CB-MCB : IOStateMachinesLib/MCB  InitSource=internal  InitState=InitState  OffStateValue=OffStateValue  OnStateValue=OnStateValue
      settings: SourceProductName=IO State Machines
  Bus Selector : BusSelector  OutputSignals=Value,Mode,InitVal,InternalRequest,Inhibit,TripRequest
  InputState : Outport  VectorParamsAs1DForOutWhenUnconnected=off
  MCBTripState : Outport  Port=2  VectorParamsAs1DForOutWhenUnconnected=off
  wires:
  AC2CB-MCB/2 -> MCBTripState/1
  Bus Selector/6 -> AC2CB-MCB/7  "<TripRequest>"
  MCBControl/1 -> Bus Selector/1
  Bus Selector/1 -> AC2CB-MCB/1  "<Value>"
  Bus Selector/2 -> AC2CB-MCB/2  "<Mode>"
  Bus Selector/3 -> AC2CB-MCB/3  "<InitVal>"
  Bus Selector/4 -> AC2CB-MCB/5  "<InternalRequest>"
  Bus Selector/5 -> AC2CB-MCB/6  "<Inhibit>"
  AC2CB-MCB/1 -> InputState/1
  Initialise/1 -> AC2CB-MCB/4

== system IOControls/ForEachVehicle/IOControls/Non-CabControl/CircuitBreakersofEDB/ADDCOS ==
  note: States:
      | Normal
      | Cutout
  InputControl : Inport  OutDataTypeStr=Bus: BD_IOControls_In_InputControl
  Initialise : Inport  Port=2
  ADDCOS-Toggle : IOStateMachinesLib/Toggle  InitSource=internal  InitState=InitState  OffStateValue=OffStateValue  OnStateValue=OnStateValue
      settings: SourceProductName=IO State Machines
  Bus Selector : BusSelector  OutputSignals=Value,Mode,InitVal,InternalRequest,Inhibit
  InputState : Outport  VectorParamsAs1DForOutWhenUnconnected=off
  wires:
  Initialise/1 -> ADDCOS-Toggle/4
  ADDCOS-Toggle/1 -> InputState/1
  Bus Selector/5 -> ADDCOS-Toggle/6  "<Inhibit>"
  Bus Selector/4 -> ADDCOS-Toggle/5  "<InternalRequest>"
  Bus Selector/3 -> ADDCOS-Toggle/3  "<InitVal>"
  Bus Selector/2 -> ADDCOS-Toggle/2  "<Mode>"
  Bus Selector/1 -> ADDCOS-Toggle/1  "<Value>"
  InputControl/1 -> Bus Selector/1

== system IOControls/ForEachVehicle/IOControls/Non-CabControl/CircuitBreakersofEDB/APSCB ==
  note: States:
      | Tripped
      | Set
  MCBControl : Inport  OutDataTypeStr=Bus: BD_IOControls_In_MCBControl
  Initialise : Inport  Port=2
  APSCB-MCB : IOStateMachinesLib/MCB  InitSource=internal  InitState=InitState  OffStateValue=OffStateValue  OnStateValue=OnStateValue
      settings: SourceProductName=IO State Machines
  Bus Selector : BusSelector  OutputSignals=Value,Mode,InitVal,InternalRequest,Inhibit,TripRequest
  InputState : Outport  VectorParamsAs1DForOutWhenUnconnected=off
  MCBTripState : Outport  Port=2  VectorParamsAs1DForOutWhenUnconnected=off
  wires:
  APSCB-MCB/2 -> MCBTripState/1
  Bus Selector/6 -> APSCB-MCB/7  "<TripRequest>"
  MCBControl/1 -> Bus Selector/1
  Bus Selector/1 -> APSCB-MCB/1  "<Value>"
  Bus Selector/2 -> APSCB-MCB/2  "<Mode>"
  Bus Selector/3 -> APSCB-MCB/3  "<InitVal>"
  Bus Selector/4 -> APSCB-MCB/5  "<InternalRequest>"
  Bus Selector/5 -> APSCB-MCB/6  "<Inhibit>"
  APSCB-MCB/1 -> InputState/1
  Initialise/1 -> APSCB-MCB/4

== system IOControls/ForEachVehicle/IOControls/Non-CabControl/CircuitBreakersofEDB/APSICB ==
  note: States:
      | Tripped
      | Set
  MCBControl : Inport  OutDataTypeStr=Bus: BD_IOControls_In_MCBControl
  Initialise : Inport  Port=2
  APSICB-MCB : IOStateMachinesLib/MCB  InitSource=internal  InitState=InitState  OffStateValue=OffStateValue  OnStateValue=OnStateValue
      settings: SourceProductName=IO State Machines
  Bus Selector : BusSelector  OutputSignals=Value,Mode,InitVal,InternalRequest,Inhibit,TripRequest
  InputState : Outport  VectorParamsAs1DForOutWhenUnconnected=off
  MCBTripState : Outport  Port=2  VectorParamsAs1DForOutWhenUnconnected=off
  wires:
  APSICB-MCB/2 -> MCBTripState/1
  Bus Selector/6 -> APSICB-MCB/7  "<TripRequest>"
  MCBControl/1 -> Bus Selector/1
  Bus Selector/1 -> APSICB-MCB/1  "<Value>"
  Bus Selector/2 -> APSICB-MCB/2  "<Mode>"
  Bus Selector/3 -> APSICB-MCB/3  "<InitVal>"
  Bus Selector/4 -> APSICB-MCB/5  "<InternalRequest>"
  Bus Selector/5 -> APSICB-MCB/6  "<Inhibit>"
  APSICB-MCB/1 -> InputState/1
  Initialise/1 -> APSICB-MCB/4

== system IOControls/ForEachVehicle/IOControls/Non-CabControl/CircuitBreakersofEDB/BCBCB ==
  note: States:
      | Tripped
      | Set
  MCBControl : Inport  OutDataTypeStr=Bus: BD_IOControls_In_MCBControl
  Initialise : Inport  Port=2
  BCBCB-MCB : IOStateMachinesLib/MCB  InitSource=internal  InitState=InitState  OffStateValue=OffStateValue  OnStateValue=OnStateValue
      settings: SourceProductName=IO State Machines
  Bus Selector : BusSelector  OutputSignals=Value,Mode,InitVal,InternalRequest,Inhibit,TripRequest
  InputState : Outport  VectorParamsAs1DForOutWhenUnconnected=off
  MCBTripState : Outport  Port=2  VectorParamsAs1DForOutWhenUnconnected=off
  wires:
  BCBCB-MCB/2 -> MCBTripState/1
  Bus Selector/6 -> BCBCB-MCB/7  "<TripRequest>"
  MCBControl/1 -> Bus Selector/1
  Bus Selector/1 -> BCBCB-MCB/1  "<Value>"
  Bus Selector/2 -> BCBCB-MCB/2  "<Mode>"
  Bus Selector/3 -> BCBCB-MCB/3  "<InitVal>"
  Bus Selector/4 -> BCBCB-MCB/5  "<InternalRequest>"
  Bus Selector/5 -> BCBCB-MCB/6  "<Inhibit>"
  BCBCB-MCB/1 -> InputState/1
  Initialise/1 -> BCBCB-MCB/4
